simulink model "motor_controller"  (R2017a)
settings: Solver=FixedStepDiscrete  StartTime=0.0  StopTime=inf  RelTol=1e-3
undefined symbols (not defined in the file or in its folder): PWMFreq
settings Model: DataTypeOverride=Off  Creator=mini  LastModifiedBy=Nicoe Welch
settings DataIOCC: SaveOutput=off  SaveTime=off
settings OptimizationCC: BlockReduction=off  ConditionallyExecuteInputs=off
settings DebuggingCC: AlgebraicLoopMsg=error  SingleTaskRateTransMsg=error
settings HardwareCC: ProdBitPerPointer=32  ProdBitPerSizeT=32  ProdBitPerPtrDiffT=32  ProdLargestAtomicFloat=None  ProdIntDivRoundTo=Undefined  ProdEndianess=Unspecified  ProdWordSize=32  ProdHWDeviceType=ASIC/FPGA->ASIC/FPGA  ProdEqTarget=off

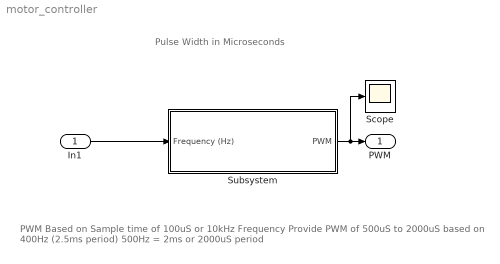
== system motor_controller ==
  note: PWM Based on Sample time of 100uS or 10kHz Frequency
      | Provide PWM of 500uS to 2000uS based on 400Hz (2.5ms period)
      | 500Hz = 2ms or 2000uS period
  note: Pulse Width in Microseconds
  In1 : Inport
  Scope : Scope
  Subsystem : Subsystem
  PWM : Outport
  wires:
  Subsystem/1(PWM) -> Scope/1, PWM/1
  In1/1 -> Subsystem/1(Frequency (Hz))

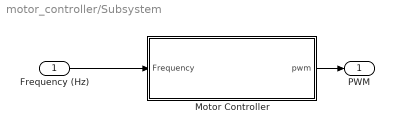
== system motor_controller/Subsystem ==
  Frequency (Hz) : Inport  OutDataTypeStr=uint32
  Motor Controller : Subsystem  mask{fpgaClk=50e6}
      mask prompts: fpgaClk "FPGA System Clock Freq"
  PWM : Outport
  wires:
  Motor Controller/1(pwm) -> PWM/1
  Frequency (Hz)/1 -> Motor Controller/1(Frequency)

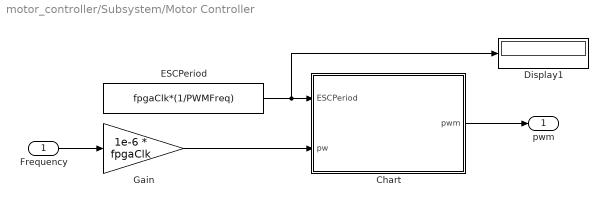
== system motor_controller/Subsystem/Motor Controller ==
  Frequency : Inport
  Chart : Stateflow chart  TreatAsAtomicUnit=on
  Display1 : Display
  ESCPeriod : Constant  Value=fpgaClk*(1/PWMFreq)  OutDataTypeStr=uint32
  Gain : Gain  Gain=1e-6 * fpgaClk  OutDataTypeStr=Inherit: Same as input
  pwm : Outport
  wires:
  Frequency/1 -> Gain/1
  Gain/1 -> Chart/2(pw)
  Chart/1(pwm) -> pwm/1
  ESCPeriod/1 -> Display1/1, Chart/1(ESCPeriod)

== stateflow chart motor_controller/Subsystem/Motor Controller/Chart ==
  settings: executeAtInitialization=1
  state on
    entry: cnt = uint32(0);
    pwm = true;
    during: cnt = cnt + 1;
  state off
    entry: pwm = false;
    during: cnt = cnt + 1;
  (default) -> on
  on -> off : [cnt > pw]
  off -> on : [cnt >= ESCPeriod]
  data: ESCPeriod input uint32; pw input uint32; pwm output boolean; cnt local uint32
